simulink library "Simple_pneu_library"  (R2017b)
settings: Solver=ode45  StartTime=0.0  StopTime=10.0  RelTol=1e-3  EnableMultiTasking=on
undefined symbols (not defined in the file or in its folder): Data, density, dsVehicleData, magnitude
settings Model: Creator=lbottazzi  LastModifiedBy=lbottazzi
settings DataIOCC: LimitDataPoints=on  SaveFormat=Array
settings OptimizationCC: LifeSpan=inf
settings DebuggingCC: SolverPrmCheckMsg=warning  SFUnexpectedBacktrackingDiag=warning  SFNoUnconditionalDefaultTransitionDiag=warning  SFExecutionAtInitializationDiag=none
settings HardwareCC: ProdBitPerPointer=32  ProdBitPerSizeT=32  ProdBitPerPtrDiffT=32  ProdLargestAtomicFloat=None  ProdIntDivRoundTo=Undefined  ProdEndianess=Unspecified  ProdWordSize=32  ProdHWDeviceType=32-bit Generic
settings ModelReferenceCC: PropagateSignalLabelsOutOfModel=off
settings CodeAppCC: StateflowObjectComments=on
settings GRTTargetCC: TargetLangStandard=C89/C90 (ANSI)  GeneratePreprocessorConditionals=Disable all
settings ConfigComp: CovMetricSettings=dw  CovHtmlReporting=on  CovSaveCumulativeToWorkspaceVar=on  CovSaveSingleToWorkspaceVar=on  CovExternalEMLEnable=off  CovSFcnEnable=off

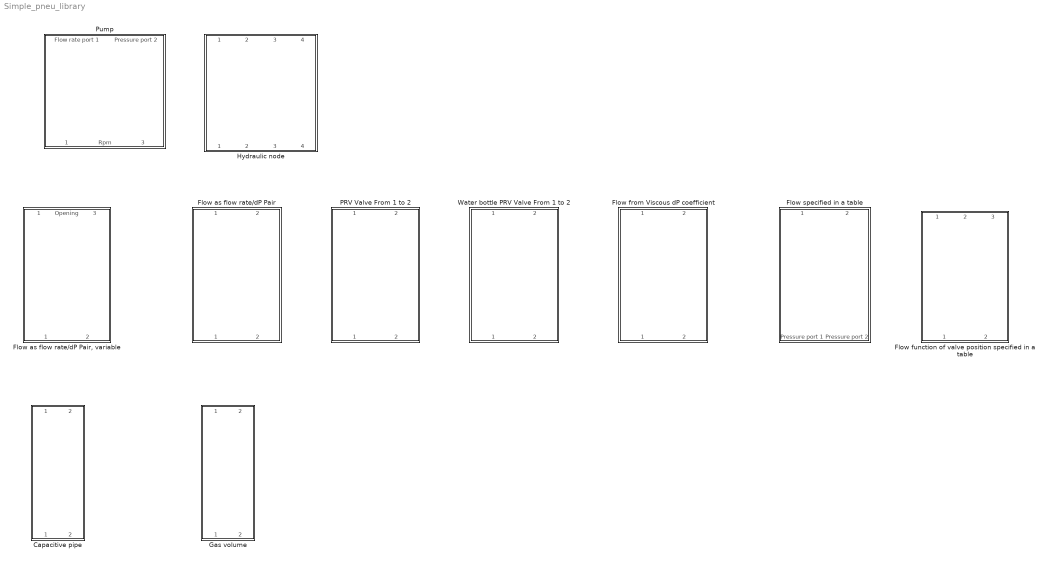
== system Simple_pneu_library ==
  Capacitive pipe : Subsystem  mask{p0=2, d=0.019, l=0.2}
      mask prompts: p0 "Initial Condition [mbar]"; d "Pipe Diameter [m]"; l "Pipe Length [m]"
  "Flow as flow rate/dP Pair, variable" : Subsystem  mask{dp=Data.XValve.dP, flow=Data.XValve.Flow}
      mask prompts: dp "Reference Pressure Drop [mbar]"; flow "Reference Flow Rate [L/min]"
  Flow as flow rate/dP Pair : Subsystem  mask{dp=5, flow=10}
      mask prompts: dp "Reference Pressure Drop [mbar]"; flow "Reference Flow Rate [L/min]"
  Flow from Viscous dP coefficient : Subsystem  mask{Viscous_losses=1}
      mask prompts: Viscous_losses "Viscous Losses [mbar/L/min]"
  Flow function of valve position specified in a table : Subsystem  mask{dp=dsVehicleData.RAD.Circuit.ENW.XValve.dP, flow=dsVehicleData.RAD.Circuit.ENW.XValve.Flow, posizione=dsVehicleData.RAD.Circuit.ENW.XValve.Position}
      mask prompts: dp "Reference Pressure Drop [mbar]"; flow "Flow Rate [L/min]"; posizione "Duty [%]"
  Flow specified in a table : Subsystem  mask{flow=Data.LHSICRadOutPipe.Flow, dp=Data.LHSICRadOutPipe.dP}
      mask prompts: flow "Flow Rate [L/min]"; dp "Pressure Drop [mbar]"
  Gas volume : Subsystem  mask{p0=2, Vol=0.019}
      mask prompts: p0 "Initial Condition [mbar]"; Vol "Volume [L]"
  Hydraulic node : Subsystem
  PRV Valve From 1 to 2 : Subsystem  mask{dp=5, flow=10, Crack=30, Delay=0.05}
      mask prompts: dp "Reference Pressure Drop [mbar]"; flow "Reference Flow Rate [L/min]"; Crack "Cracking pressure [mbar]"; Delay "Time constant for valve delay"
  Pump : Subsystem  mask{rpm=Data.Pump.Breakpoint.RPM, flow=Data.Pump.Breakpoint.Flow, dp=Data.Pump.dP, hz=100}
      mask prompts: rpm "Pump Speed [rpm]"; flow "Flow Rate [L/min]"; dp "Pressure Drop [mbar]"; hz "Filter Frequency [Hz]"
  Water bottle PRV Valve From 1 to 2 : Subsystem  mask{Viscous_losses=0.1, Crack=30, Delay=0.001}
      mask prompts: Viscous_losses "Viscous Losses [mbar/L/min]"; Crack "Cracking pressure [mbar]"; Delay "Time constant for valve delay"

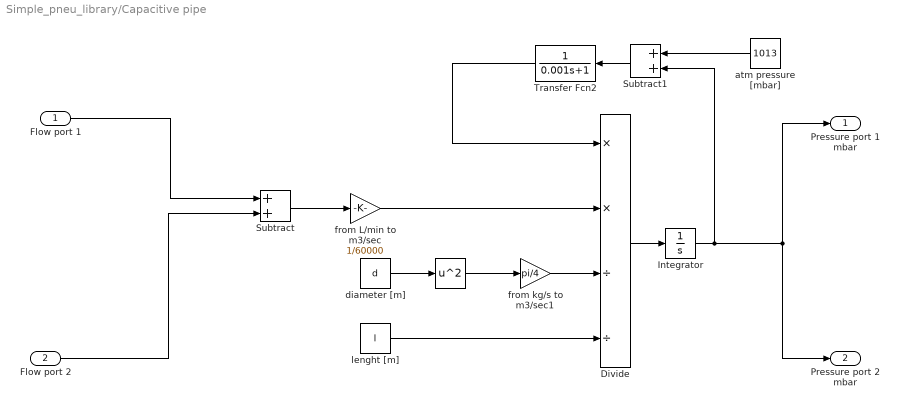
== system Simple_pneu_library/Capacitive pipe ==
  Flow port 1 : Inport
  Flow port 2 : Inport  Port=2
  " " : Math  Operator=square  SaturateOnIntegerOverflow=on
  Divide : Product  Inputs=**//
  Integrator : Integrator  InitialCondition=p0  ZeroCross=off
  Subtract : Sum
  Subtract1 : Sum
  Transfer Fcn2 : TransferFcn  Denominator=[0.001 1]
  atm pressure [mbar] : Constant  Value=1013
  diameter [m] : Constant  Value=d
  from L/min to m3/sec : Gain  Gain=1/60000
  from kg/s to m3/sec1 : Gain  Gain=pi/4
  lenght [m] : Constant  Value=l
  Pressure port 1 mbar : Outport
  Pressure port 2 mbar : Outport  Port=2
  wires:
  from kg/s to m3/sec1/1 -> Divide/3
  " "/1 -> from kg/s to m3/sec1/1
  Subtract/1 -> from L/min to m3/sec/1
  from L/min to m3/sec/1 -> Divide/2
  Divide/1 -> Integrator/1
  lenght [m]/1 -> Divide/4
  diameter [m]/1 -> " "/1
  Flow port 1/1 -> Subtract/1
  Flow port 2/1 -> Subtract/2
  Integrator/1 -> Subtract1/2, Pressure port 2 mbar/1, Pressure port 1 mbar/1
  Subtract1/1 -> Transfer Fcn2/1
  atm pressure [mbar]/1 -> Subtract1/1
  Transfer Fcn2/1 -> Divide/1

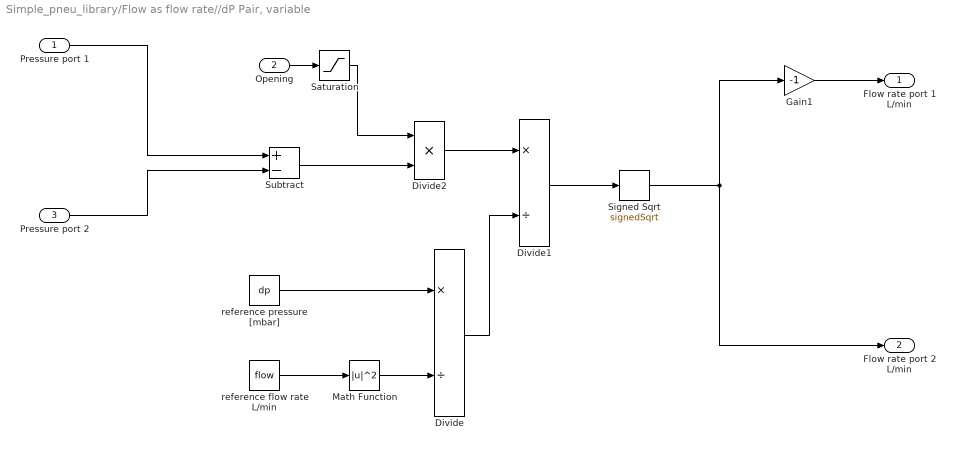
== system Simple_pneu_library/Flow as flow rate//dP Pair, variable ==
  "Pressure port 1 " : Inport
  Opening : Inport  Port=2
  "Pressure port 2 " : Inport  Port=3
  Divide : Product  Inputs=*/
  Divide1 : Product  Inputs=*/
  Divide2 : Product  Inputs=**
  Gain1 : Gain  Gain=-1
  Math Function : Math  Operator=magnitude^2  SaturateOnIntegerOverflow=on
  Saturation : Saturate  UpperLimit=1  LowerLimit=0
  Signed Sqrt : Sqrt  Operator=signedSqrt  SaturateOnIntegerOverflow=on
  Subtract : Sum  Inputs=+-
  reference flow rate L/min : Constant  Value=flow
  reference pressure [mbar] : Constant  Value=dp
  "Flow rate port 1 L/min " : Outport
  "Flow rate port 2 L/min " : Outport  Port=2
  wires:
  Signed Sqrt/1 -> Gain1/1, "Flow rate port 2 L/min "/1
  Divide1/1 -> Signed Sqrt/1
  Divide/1 -> Divide1/2
  reference pressure [mbar]/1 -> Divide/1
  Math Function/1 -> Divide/2
  Gain1/1 -> "Flow rate port 1 L/min "/1
  "Pressure port 1 "/1 -> Subtract/1
  "Pressure port 2 "/1 -> Subtract/2
  Opening/1 -> Saturation/1
  Saturation/1 -> Divide2/1
  Divide2/1 -> Divide1/1
  Subtract/1 -> Divide2/2
  reference flow rate L/min/1 -> Math Function/1

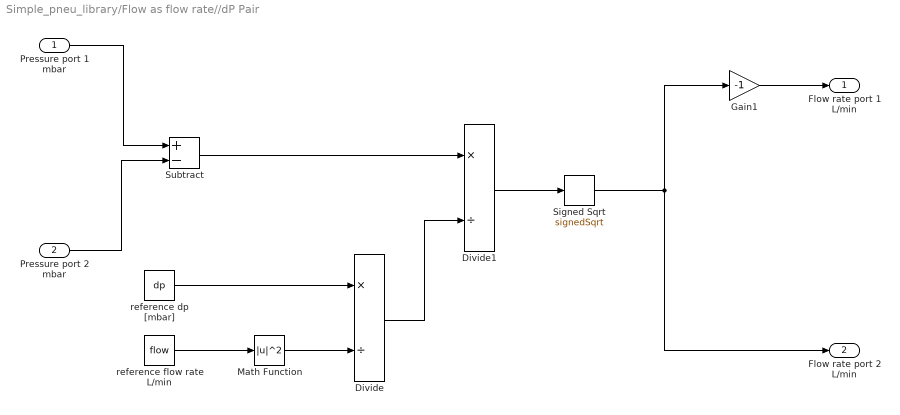
== system Simple_pneu_library/Flow as flow rate//dP Pair ==
  "Pressure port 1 mbar " : Inport
  "Pressure port 2 mbar " : Inport  Port=2
  Divide : Product  Inputs=*/
  Divide1 : Product  Inputs=*/
  Gain1 : Gain  Gain=-1
  Math Function : Math  Operator=magnitude^2  SaturateOnIntegerOverflow=on
  Signed Sqrt : Sqrt  Operator=signedSqrt  SaturateOnIntegerOverflow=on
  Subtract : Sum  Inputs=+-
  reference dp [mbar] : Constant  Value=dp
  reference flow rate L/min : Constant  Value=flow
  "Flow rate port 1 L/min " : Outport
  "Flow rate port 2 L/min " : Outport  Port=2
  wires:
  "Pressure port 2 mbar "/1 -> Subtract/2
  "Pressure port 1 mbar "/1 -> Subtract/1
  Subtract/1 -> Divide1/1
  Gain1/1 -> "Flow rate port 1 L/min "/1
  reference flow rate L/min/1 -> Math Function/1
  Math Function/1 -> Divide/2
  reference dp [mbar]/1 -> Divide/1
  Divide/1 -> Divide1/2
  Divide1/1 -> Signed Sqrt/1
  Signed Sqrt/1 -> "Flow rate port 2 L/min "/1, Gain1/1

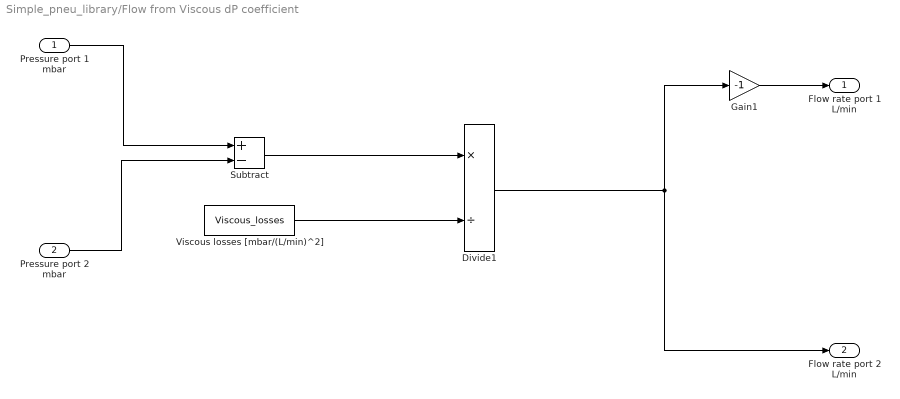
== system Simple_pneu_library/Flow from Viscous dP coefficient ==
  "Pressure port 1 mbar " : Inport
  "Pressure port 2 mbar " : Inport  Port=2
  Divide1 : Product  Inputs=*/
  Gain1 : Gain  Gain=-1
  Subtract : Sum  Inputs=+-
  Viscous losses [mbar/(L/min)^2] : Constant  Value=Viscous_losses
  "Flow rate port 1 L/min " : Outport
  "Flow rate port 2 L/min " : Outport  Port=2
  wires:
  "Pressure port 2 mbar "/1 -> Subtract/2
  "Pressure port 1 mbar "/1 -> Subtract/1
  Subtract/1 -> Divide1/1
  Gain1/1 -> "Flow rate port 1 L/min "/1
  Viscous losses [mbar/(L/min)^2]/1 -> Divide1/2
  Divide1/1 -> "Flow rate port 2 L/min "/1, Gain1/1

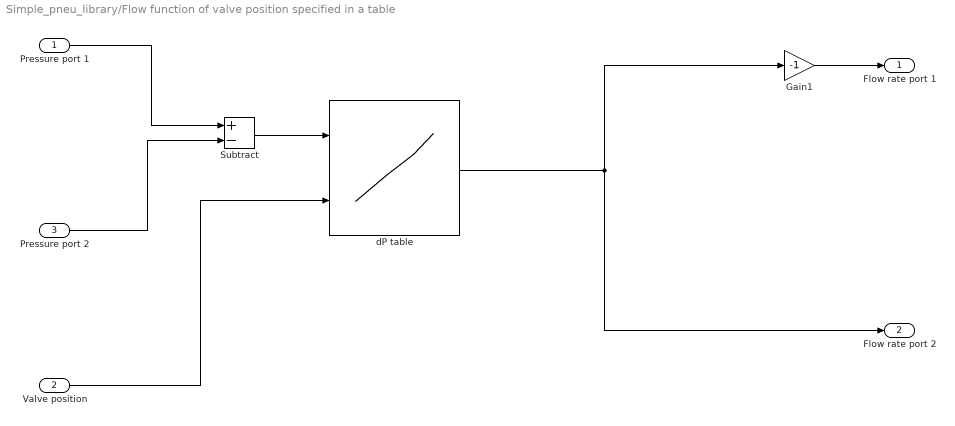
== system Simple_pneu_library/Flow function of valve position specified in a table ==
  "Pressure port 1 " : Inport
  Valve position : Inport  Port=2
  Pressure port 2 : Inport  Port=3
  Gain1 : Gain  Gain=-1
  Subtract : Sum  Inputs=+-
  dP table : Lookup_n-D  BreakpointsForDimension1=dp  BreakpointsForDimension2=posizione  BeginIndexSearchUsingPreviousIndexResult=on  Table=flow  InterpMethod=Cubic spline  InternalRulePriority=Speed  RndMeth=Simplest  InputSameDT=on
  "Flow rate port 1 " : Outport
  "Flow rate port 2 " : Outport  Port=2
  wires:
  "Pressure port 1 "/1 -> Subtract/1
  Subtract/1 -> dP table/1
  Gain1/1 -> "Flow rate port 1 "/1
  Pressure port 2/1 -> Subtract/2
  Valve position/1 -> dP table/2
  dP table/1 -> "Flow rate port 2 "/1, Gain1/1

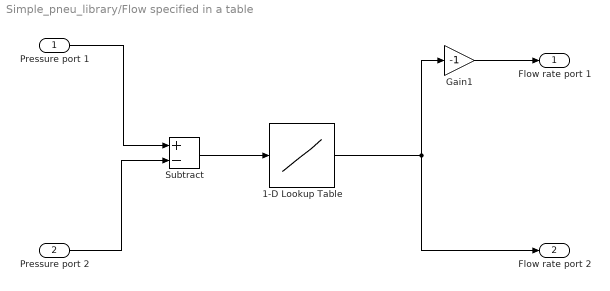
== system Simple_pneu_library/Flow specified in a table ==
  "Pressure port 1 " : Inport
  "Pressure port 2 " : Inport  Port=2
  1-D Lookup Table : Lookup_n-D  NumberOfTableDimensions=1  BreakpointsForDimension1=dp  BeginIndexSearchUsingPreviousIndexResult=on  Table=flow  InterpMethod=Cubic spline  InternalRulePriority=Speed  RndMeth=Simplest  InputSameDT=on
  Gain1 : Gain  Gain=-1
  Subtract : Sum  Inputs=+-
  "Flow rate port 1 " : Outport
  "Flow rate port 2 " : Outport  Port=2
  wires:
  "Pressure port 2 "/1 -> Subtract/2
  "Pressure port 1 "/1 -> Subtract/1
  Subtract/1 -> 1-D Lookup Table/1
  Gain1/1 -> "Flow rate port 1 "/1
  1-D Lookup Table/1 -> "Flow rate port 2 "/1, Gain1/1

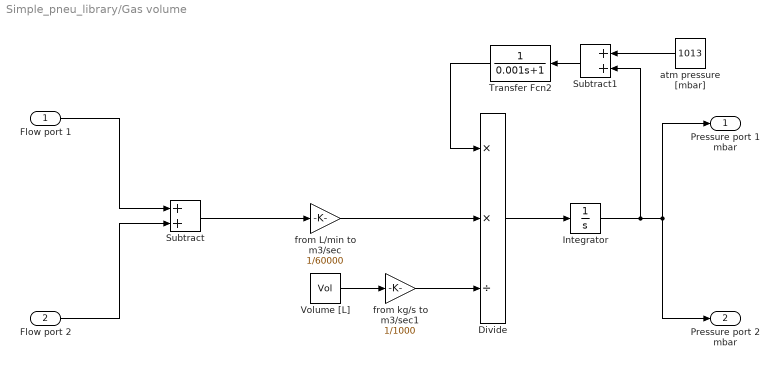
== system Simple_pneu_library/Gas volume ==
  Flow port 1 : Inport
  Flow port 2 : Inport  Port=2
  Divide : Product  Inputs=**/
  Integrator : Integrator  InitialCondition=p0  ZeroCross=off
  Subtract : Sum
  Subtract1 : Sum
  Transfer Fcn2 : TransferFcn  Denominator=[0.001 1]
  Volume [L] : Constant  Value=Vol
  atm pressure [mbar] : Constant  Value=1013
  from L/min to m3/sec : Gain  Gain=1/60000
  from kg/s to m3/sec1 : Gain  Gain=1/1000
  Pressure port 1 mbar : Outport
  Pressure port 2 mbar : Outport  Port=2
  wires:
  Flow port 2/1 -> Subtract/2
  Flow port 1/1 -> Subtract/1
  Volume [L]/1 -> from kg/s to m3/sec1/1
  Integrator/1 -> Subtract1/2, Pressure port 2 mbar/1, Pressure port 1 mbar/1
  Divide/1 -> Integrator/1
  from L/min to m3/sec/1 -> Divide/2
  Subtract/1 -> from L/min to m3/sec/1
  from kg/s to m3/sec1/1 -> Divide/3
  Transfer Fcn2/1 -> Divide/1
  Subtract1/1 -> Transfer Fcn2/1
  atm pressure [mbar]/1 -> Subtract1/1

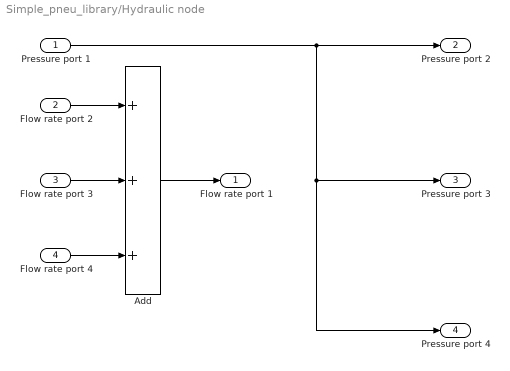
== system Simple_pneu_library/Hydraulic node ==
  "Pressure port 1 " : Inport
  Flow rate port 2 : Inport  Port=2
  Flow rate port 3 : Inport  Port=3
  Flow rate port 4 : Inport  Port=4
  Add : Sum  Inputs=+++
  "Flow rate port 1 " : Outport
  Pressure port 2 : Outport  Port=2
  Pressure port 3 : Outport  Port=3
  Pressure port 4 : Outport  Port=4
  wires:
  "Pressure port 1 "/1 -> Pressure port 4/1, Pressure port 3/1, Pressure port 2/1
  Add/1 -> "Flow rate port 1 "/1
  Flow rate port 2/1 -> Add/1
  Flow rate port 3/1 -> Add/2
  Flow rate port 4/1 -> Add/3

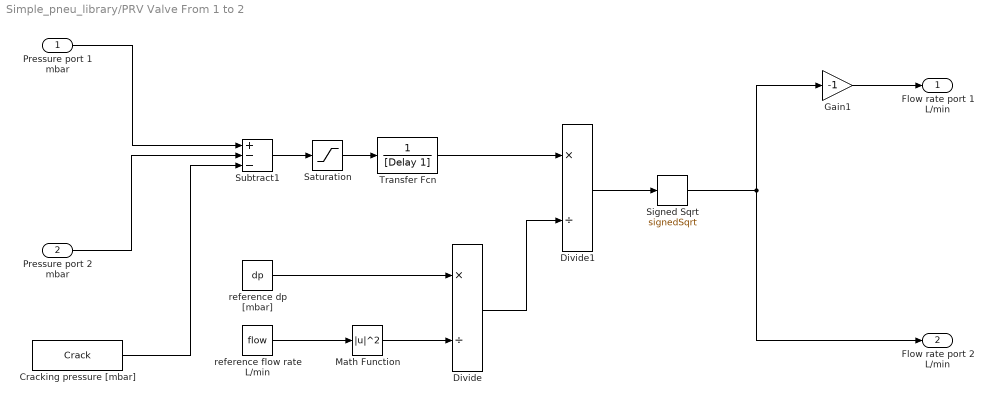
== system Simple_pneu_library/PRV Valve From 1 to 2 ==
  "Pressure port 1 mbar " : Inport
  "Pressure port 2 mbar " : Inport  Port=2
  Cracking pressure [mbar] : Constant  Value=Crack
  Divide : Product  Inputs=*/
  Divide1 : Product  Inputs=*/
  Gain1 : Gain  Gain=-1
  Math Function : Math  Operator=magnitude^2  SaturateOnIntegerOverflow=on
  Saturation : Saturate  UpperLimit=1e10  LowerLimit=0
  Signed Sqrt : Sqrt  Operator=signedSqrt  SaturateOnIntegerOverflow=on
  Subtract1 : Sum  Inputs=+--
  Transfer Fcn : TransferFcn  Denominator=[Delay 1]
  reference dp [mbar] : Constant  Value=dp
  reference flow rate L/min : Constant  Value=flow
  "Flow rate port 1 L/min " : Outport
  "Flow rate port 2 L/min " : Outport  Port=2
  wires:
  Signed Sqrt/1 -> "Flow rate port 2 L/min "/1, Gain1/1
  Divide1/1 -> Signed Sqrt/1
  Divide/1 -> Divide1/2
  reference dp [mbar]/1 -> Divide/1
  Math Function/1 -> Divide/2
  reference flow rate L/min/1 -> Math Function/1
  Gain1/1 -> "Flow rate port 1 L/min "/1
  "Pressure port 1 mbar "/1 -> Subtract1/1
  "Pressure port 2 mbar "/1 -> Subtract1/2
  Cracking pressure [mbar]/1 -> Subtract1/3
  Subtract1/1 -> Saturation/1
  Saturation/1 -> Transfer Fcn/1
  Transfer Fcn/1 -> Divide1/1

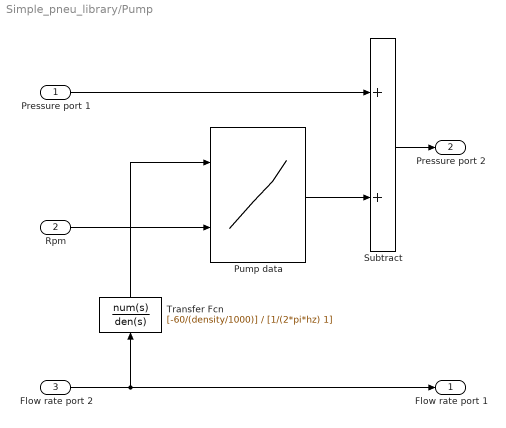
== system Simple_pneu_library/Pump ==
  "Pressure port 1 " : Inport
  Rpm : Inport  Port=2
  Flow rate port 2 : Inport  Port=3
  Pump data : Lookup_n-D  BreakpointsForDimension1=flow  BreakpointsForDimension2=rpm  BeginIndexSearchUsingPreviousIndexResult=on  Table=dp  ExtrapMethod=Clip  InternalRulePriority=Speed  RndMeth=Simplest  InputSameDT=on
  Subtract : Sum
  Transfer Fcn : TransferFcn  Numerator=[-60/(density/1000)]  Denominator=[1/(2*pi*hz) 1]
  "Flow rate port 1 " : Outport
  Pressure port 2 : Outport  Port=2
  wires:
  Flow rate port 2/1 -> "Flow rate port 1 "/1, Transfer Fcn/1
  Pump data/1 -> Subtract/2
  Subtract/1 -> Pressure port 2/1
  "Pressure port 1 "/1 -> Subtract/1
  Rpm/1 -> Pump data/2
  Transfer Fcn/1 -> Pump data/1

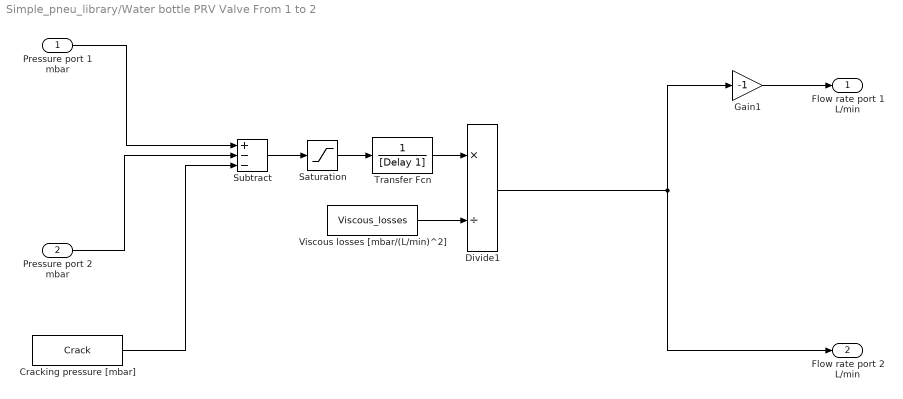
== system Simple_pneu_library/Water bottle PRV Valve From 1 to 2 ==
  "Pressure port 1 mbar " : Inport
  "Pressure port 2 mbar " : Inport  Port=2
  Cracking pressure [mbar] : Constant  Value=Crack
  Divide1 : Product  Inputs=*/
  Gain1 : Gain  Gain=-1
  Saturation : Saturate  UpperLimit=1e10  LowerLimit=0
  Subtract : Sum  Inputs=+--
  Transfer Fcn : TransferFcn  Denominator=[Delay 1]
  Viscous losses [mbar/(L/min)^2] : Constant  Value=Viscous_losses
  "Flow rate port 1 L/min " : Outport
  "Flow rate port 2 L/min " : Outport  Port=2
  wires:
  Divide1/1 -> Gain1/1, "Flow rate port 2 L/min "/1
  Viscous losses [mbar/(L/min)^2]/1 -> Divide1/2
  Gain1/1 -> "Flow rate port 1 L/min "/1
  "Pressure port 1 mbar "/1 -> Subtract/1
  "Pressure port 2 mbar "/1 -> Subtract/2
  Cracking pressure [mbar]/1 -> Subtract/3
  Subtract/1 -> Saturation/1
  Saturation/1 -> Transfer Fcn/1
  Transfer Fcn/1 -> Divide1/1
